simulink model "pr11"  (Simulink 7.5)
settings: Solver=ode45  StartTime=0.0  StopTime=1  RelTol=1e-3
settings Model: Creator=Fer  LastModifiedBy=Fer

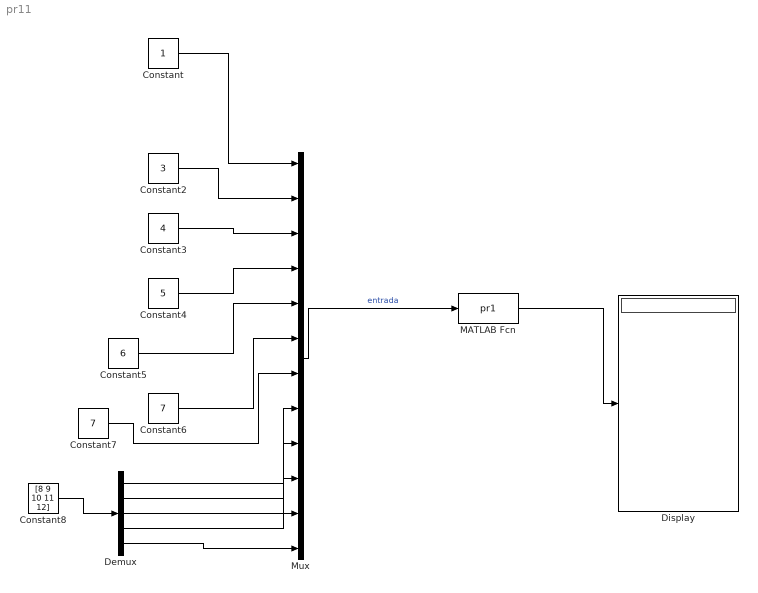
== system pr11 ==
  Constant : Constant  OutDataType=fixdt(1, 16)  OutScaling=2^0
  Constant2 : Constant  Value=3  OutDataType=fixdt(1, 16)  OutScaling=2^0
  Constant3 : Constant  Value=4  OutDataType=fixdt(1, 16)  OutScaling=2^0
  Constant4 : Constant  Value=5  OutDataType=fixdt(1, 16)  OutScaling=2^0
  Constant5 : Constant  Value=6  OutDataType=fixdt(1, 16)  OutScaling=2^0
  Constant6 : Constant  Value=7  OutDataType=fixdt(1, 16)  OutScaling=2^0
  Constant7 : Constant  Value=7  OutDataType=fixdt(1, 16)  OutScaling=2^0
  Constant8 : Constant  Value=[8 9 10 11 12]  OutDataType=fixdt(1, 16)  OutScaling=2^0
  Demux : Demux  Outputs=5
  Display : Display
  MATLAB Fcn : MATLABFcn  MATLABFcn=pr1
  Mux : Mux  Inputs=12
  wires:
  Constant/1 -> Mux/1
  Mux/1 -> MATLAB Fcn/1  "entrada"
  MATLAB Fcn/1 -> Display/1
  Constant2/1 -> Mux/2
  Constant3/1 -> Mux/3
  Constant4/1 -> Mux/4
  Constant5/1 -> Mux/5
  Constant6/1 -> Mux/6
  Constant7/1 -> Mux/7
  Constant8/1 -> Demux/1
  Demux/1 -> Mux/8
  Demux/2 -> Mux/9
  Demux/3 -> Mux/10
  Demux/4 -> Mux/11
  Demux/5 -> Mux/12
